simulink model "new_Sim_Simulink"  (R2022a)
settings: Solver=FixedStepAuto  StartTime=0.0  StopTime=tf  FixedStep=dt  RelTol=1e-3
values from neighbouring files (symbols this model uses):
  Desired = 2    [project_code.m]
  K = k_bar(1:4)    [project_code.m]
  K2 = k_bar(5)    [project_code.m]
  Model = 1    [project_code.m]
  x_initial = [-0.5 ; 0 ; deg2rad(30) ; 0]    [project_code.m]
  xd = [0.5 , 0 , 0 , 0]    [project_code.m]
settings Model: Creator=brendoncallen  LastModifiedBy=anw0060
settings SolverCC: AlgebraicLoopSolver=TrustRegion
settings DataIOCC: ReturnWorkspaceOutputs=off
settings DebuggingCC: UnconnectedInputMsg=warning  UnconnectedOutputMsg=warning  UnconnectedLineMsg=warning  SFMachineParentedDataDiag=warning  ArithmeticOperatorsInVariantConditions=warning
settings SFSimCC: SimUseLocalCustomCode=off  CustomCodeUndefinedFunction=UseInterfaceOnly
settings RTWCC: RTWUseLocalCustomCode=off  DLArmComputeVersion=19.05

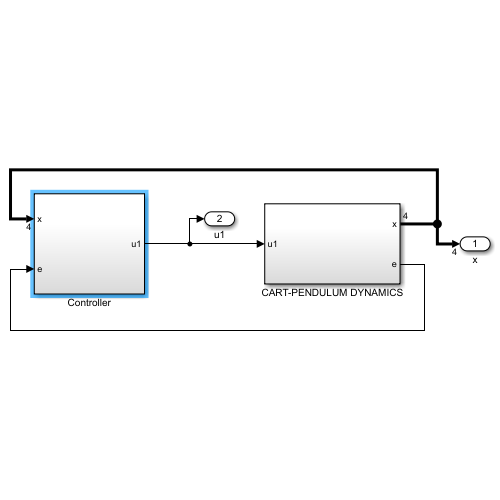
[thumbnail: Simulink's stored preview of the top-level diagram]
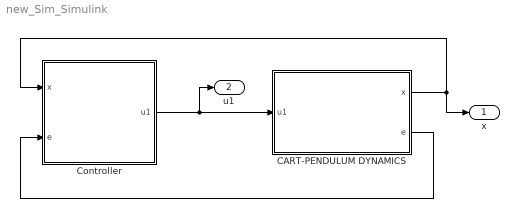
== system new_Sim_Simulink ==
  CART-PENDULUM DYNAMICS : Subsystem
  Controller : Subsystem
  x : Outport  VectorParamsAs1DForOutWhenUnconnected=off
  u1 : Outport  Port=2  VectorParamsAs1DForOutWhenUnconnected=off
  wires:
  CART-PENDULUM DYNAMICS/1(x) -> x/1, Controller/1(x)
  Controller/1(u1) -> u1/1, CART-PENDULUM DYNAMICS/1(u1)
  CART-PENDULUM DYNAMICS/2(e) -> Controller/2(e)

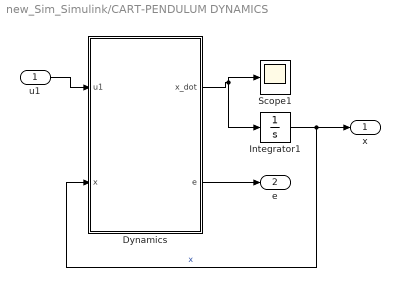
== system new_Sim_Simulink/CART-PENDULUM DYNAMICS ==
  u1 : Inport
  Dynamics : MATLAB Function  TreatAsAtomicUnit=on
  Integrator1 : Integrator  InitialCondition=x_initial
  Scope1 : Scope
  x : Outport  VectorParamsAs1DForOutWhenUnconnected=off
  e : Outport  Port=2
  wires:
  Dynamics/1(x_dot) -> Scope1/1, Integrator1/1
  Integrator1/1 -> x/1, Dynamics/2(x)  "x"
  u1/1 -> Dynamics/1(u1)
  Dynamics/2(e) -> e/1

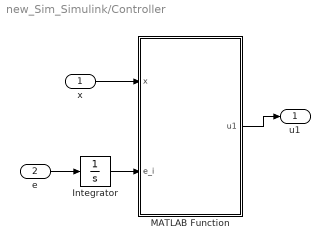
== system new_Sim_Simulink/Controller ==
  x : Inport
  e : Inport  Port=2
  Integrator : Integrator
  MATLAB Function : MATLAB Function  TreatAsAtomicUnit=on
  u1 : Outport  VectorParamsAs1DForOutWhenUnconnected=off
  wires:
  x/1 -> MATLAB Function/1(x)
  MATLAB Function/1(u1) -> u1/1
  e/1 -> Integrator/1
  Integrator/1 -> MATLAB Function/2(e_i)

== matlab function new_Sim_Simulink/Controller/MATLAB Function ==
  data: x input size=4; u1 output size=1; K parameter; Desired parameter; K2 parameter; e_i input
function u1 = controller(x, K , Desired,K2,e_i)

if Desired==1
    u1 = -K*x;
else
    u1=-K*x-K2*e_i;
end

end

== matlab function new_Sim_Simulink/CART-PENDULUM DYNAMICS/Dynamics ==
  data: u1 input size=1; x input size=4; x_dot output size=4; Model parameter size=1; e output; xd parameter
function [x_dot, e] = dynamics(u1,x,Model, xd)

% Inverted Pendulum-Cart System

%   x is the state vector of [x; x_dot; phi; phi_dot],  4x1 vector
%   u is the control input the the cart,                1x1 scalar
%   phi is measured from the upward vertical in the CCW direction.
%   u is the control input in the positive right direction
%   x is measured relative to a desired x-cooridnate

%% System Parameters
M = 0.5;     %Mass of the Cart [kg]
m = 0.2;     %Mass of the pendulum [kg]
b = 0.1;     %Coeff of friction for the cart
l = 0.3;     %Length to pendulum CoM
I = 0.006;   %Moment of inertia of the pendulum
g = 9.8;  %Gravitational Const. [m/s^2]

ml = m*l; % To reduce # of calculations

%% System Model

x1 = x(1);
x2 = x(2);
x3 = x(3);
x4 = x(4);

if Model == 1 %Linear Model
   
    a1=M*l^2*m+I*M+I*m;
    A = [0 , 1 , 0 , 0; ... 
        0 , (-I*b-b*l^2*m)/a1 , (m^2*g*l^2)/a1 , 0; ...
        0 , 0 , 0 , 1; ...
        0 , (-b*l*m)/a1 , (M*g*l*m+m^2*g*l)/a1 , 0];
    B = [0 ; (I+l^2*m)/a1 ; 0 ; (l*m)/a1];

    x_dot = A*x + B*u1;
else % Nonlinear Model


    x_dot_1 = x2;
    x_dot_2 = -((I*b*x2-u1*I-u1*(l^2)*m+b*(l^2)*m*x2+(l^3)*(m^2)*(x4^2)*sin(x3)-g*(l^2)*(m^2)*cos(x3)*sin(x3)+I*l*m*(x4^2)*sin(x3))/(-(l^2)*(m^2)*(cos(x3)^2)+(l^2)*(m^2)+M*(l^2)*m+I*m+I*m));
    x_dot_3 = x4;
    x_dot_4 = (l*m*(-l*m*cos(x3)*sin(x3)*(x4^2)+u1*cos(x3)+M*g*sin(x3)-b*x2*cos(x3)+g*m*sin(x3)))/(-(l^2)*(m^2)*(cos(x3)^2)+(l^2)*(m^2)+M*(l^2)*m+I*m+I*m);

    x_dot = [x_dot_1;x_dot_2;x_dot_3;x_dot_4];

    
end
e = x1 - xd(1);

end
